simulink model "basic_DTC_model"  (R2024b)
settings: Solver=ode23tb  StartTime=0.0  StopTime=0.4  RelTol=1e-3
InitFcn:
  | pn = 4;
  | Ld = 8.5e-3;
  | Lq = 8.5e-3;
  | R = 1.2;
  | phi = 0.175;
  | J = 0.0008;
  | B = 0.000;
libraries: spsGroundLib x1, spsUniversalBridgeLib x1, spsPermanentMagnetSynchronousMachineLib x1, spsThreePhaseVIMeasurementLib x1, spsDCVoltageSourceLib x1, sps_lib x1

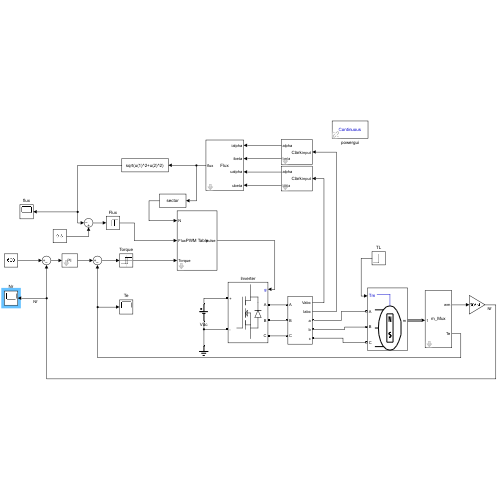
[thumbnail: Simulink's stored preview of the top-level diagram]
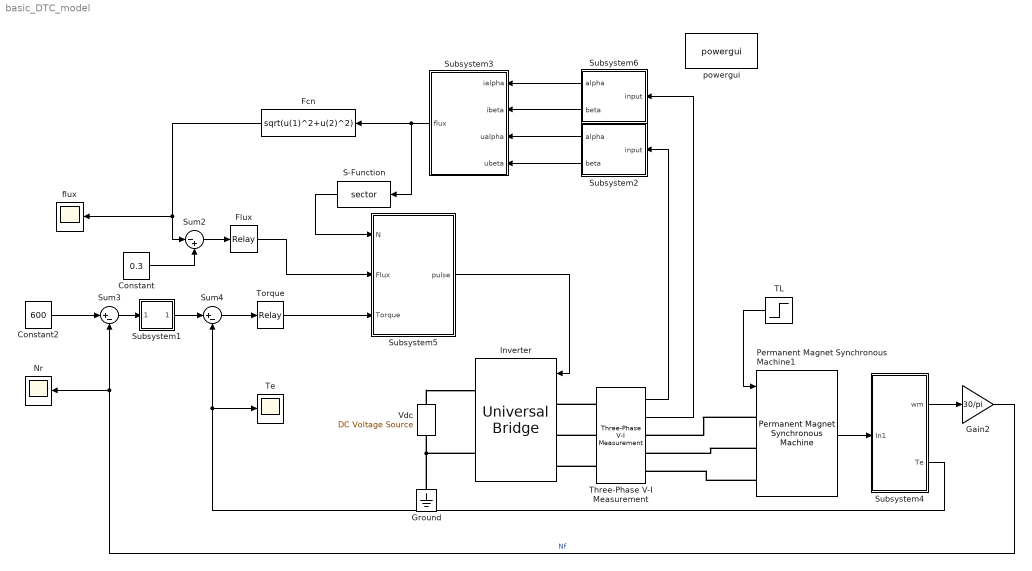
== system basic_DTC_model ==
  Constant : Constant  Value=0.3
  Constant2 : Constant  Value=600
  Fcn : Fcn  Expr=sqrt(u(1)^2+u(2)^2)
  Flux : Relay  OnSwitchValue=0.002  OffSwitchValue=-0.002
  Gain2 : Gain  Gain=30/pi
  Ground : spsGroundLib/Ground  LConnTagsString=a
  Inverter : spsUniversalBridgeLib/Universal Bridge  Arms=3  SnubberResistance=1e5  SnubberCapacitance=inf  Device=MOSFET / Diodes  Ron=1e-3  Lon=0  ForwardVoltages="[  0  0  ]"  ForwardVoltage=0  GTOparameters=[ 10e-6 , 20e-6 ]  IGBTparameters=[ 1e-6 , 2e-6 ]  Measurements=None  Measurements_2=None  converterType=Rectifier
  Nr : Scope
  Permanent Magnet Synchronous Machine1 : spsPermanentMagnetSynchronousMachineLib/Permanent Magnet Synchronous Machine  NbPhases=3  FluxDistribution=Sinusoidal  RotorType=Salient-pole  MechanicalLoad=Torque Tm  PresetModel=No  ShowDetailedParameters=on  MeasurementBus=off  Resistance=R  Inductance=8.5e-3  dqInductances=[Ld Lq]  La=0.000395  MachineConstant=Flux linkage established by magnets (V.s)  Flux=phi  VoltageCst=132.5525  TorqueCst=1.0962  Flat=120  Mechanical=[J B pn 0]  PolePairs=2  InitialConditions=[0,0, 0,0]  InitialConditions5ph=[0 0 0 0 0 0]  RefAngle=Aligned with phase A axis (original Park)  IterativeDiscreteModel=Trapezoidal non iterative  TsBlock=-1  TsPowergui=0
  S-Function : S-Function  FunctionName=sector  SFunctionModules='sector'  SFunctionDeploymentMode=off  EnableBusSupport=off
  Subsystem1 : Subsystem
  Subsystem2 : Subsystem
  Subsystem3 : Subsystem
  Subsystem4 : Subsystem
  Subsystem5 : Subsystem
  Subsystem6 : Subsystem
  Sum2 : Sum  Inputs=|-+
  Sum3 : Sum  Inputs=|+-
  Sum4 : Sum  Inputs=|+-
  TL : Step  Time=0.2  After=1.5  SampleTime=0
  Te : Scope
  Three-Phase V-I Measurement : spsThreePhaseVIMeasurementLib/Three-Phase V-I Measurement  VoltageMeasurement=phase-to-ground  SetLabelV=off  LabelV=Vabc  Vpu=off  VpuLL=off  CurrentMeasurement=yes  SetLabelI=off  LabelI=Iabc  Ipu=off  Pbase=100e6  Vbase=500e3  OutputType=Complex  PhasorSimulation=off  PSBequivalent=0
  Torque : Relay  OnSwitchValue=0.1  OffSwitchValue=-0.1
  Vdc : spsDCVoltageSourceLib/DC Voltage Source  Amplitude=311  Measurements=None
  flux : Scope
  powergui : sps_lib/powergui  Priority=1  SimulationMode=Continuous  SampleTime=10e-6  frequency=60  Iterations=50  frequencyindice=0  Pbase=100e6  ErrMax=1e-4  UnitsV=kV  UnitsW=MW  buscounter=0  FunctionMessages=off  echomessages=off  EnableUseOfTLC=off  CurrentSourceSwitches=off  DisableSnubberDevices=off  DisableRonSwitches=off  DisableVfSwitches=off  DisplayEquations=off  AutomaticDiscreteSolvers=off  SolverType=Tustin/Backward Euler (TBE)  Interpol=off  ExternalGateDelay=off  methode=off  Ts=100  x0status=blocks  SPID=on  SwTol=0  HookPort=off  NonlinearTolerance=1e-4  nMaxIteration=100  ContinueOnMaxIteration=off  RestoreLinks=warning  ResistiveCurrentMeasurement=off  Frange=[0:2:500]  Ylog=off  Xlog=on  ShowGrid=off  save=off  variable=ZData  structure=0  ZoomFFT=off  StartTime=0.0  cycles=1  DisplayStyle=1  fundamental=60  FreqAxis=off  MaxFrequency=1000  frequencyindicesteady=1  RmsSteady=1  display=off
  wires:
  TL/1 -> Permanent Magnet Synchronous Machine1/1
  Permanent Magnet Synchronous Machine1/1 -> Subsystem4/1(In1)
  Subsystem4/2(Te) -> Sum4/2, Te/1
  Subsystem5/1(pulse) -> Inverter/1
  Constant2/1 -> Sum3/1
  Sum3/1 -> Subsystem1/1(Input)
  Subsystem3/1(flux) -> S-Function/1, Fcn/1
  Constant/1 -> Sum2/2
  Fcn/1 -> flux/1, Sum2/1
  S-Function/1 -> Subsystem5/1(N)
  Sum2/1 -> Flux/1
  Flux/1 -> Subsystem5/2(Flux)
  Sum4/1 -> Torque/1
  Subsystem1/1(output) -> Sum4/1
  Torque/1 -> Subsystem5/3(Torque)
  Subsystem4/1(wm) -> Gain2/1
  Gain2/1 -> Sum3/2, Nr/1  "Nf"
  Three-Phase V-I Measurement/1 -> Subsystem2/1(input)
  Subsystem2/1(alpha) -> Subsystem3/3(ualpha)
  Subsystem2/2(beta) -> Subsystem3/4(ubeta)
  Subsystem6/2(beta) -> Subsystem3/2(ibeta)
  Subsystem6/1(alpha) -> Subsystem3/1(ialpha)
  Three-Phase V-I Measurement/2 -> Subsystem6/1(input)
  connections:
  Vdc/RConn1 -- Inverter/RConn1
  Inverter/RConn2 -- Ground/LConn1 -- Vdc/LConn1
  Three-Phase V-I Measurement/LConn1 -- Inverter/LConn1
  Three-Phase V-I Measurement/LConn2 -- Inverter/LConn2
  Three-Phase V-I Measurement/LConn3 -- Inverter/LConn3
  Permanent Magnet Synchronous Machine1/LConn1 -- Three-Phase V-I Measurement/RConn1
  Permanent Magnet Synchronous Machine1/LConn2 -- Three-Phase V-I Measurement/RConn2
  Permanent Magnet Synchronous Machine1/LConn3 -- Three-Phase V-I Measurement/RConn3

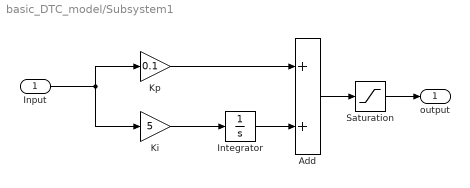
== system basic_DTC_model/Subsystem1 ==
  Input : Inport
  Add : Sum
  Integrator : Integrator
  Ki : Gain  Gain=5
  Kp : Gain  Gain=0.1
  Saturation : Saturate  UpperLimit=5  LowerLimit=-5
  output : Outport
  wires:
  Input/1 -> Ki/1, Kp/1
  Ki/1 -> Integrator/1
  Integrator/1 -> Add/2
  Kp/1 -> Add/1
  Add/1 -> Saturation/1
  Saturation/1 -> output/1

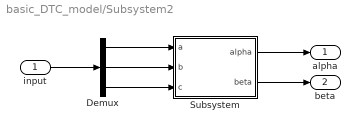
== system basic_DTC_model/Subsystem2 ==
  input : Inport
  Demux : Demux  Outputs=3
  Subsystem : Subsystem
  alpha : Outport
  beta : Outport  Port=2
  wires:
  input/1 -> Demux/1
  Demux/1 -> Subsystem/1(a)
  Demux/2 -> Subsystem/2(b)
  Demux/3 -> Subsystem/3(c)
  Subsystem/1(alpha) -> alpha/1
  Subsystem/2(beta) -> beta/1

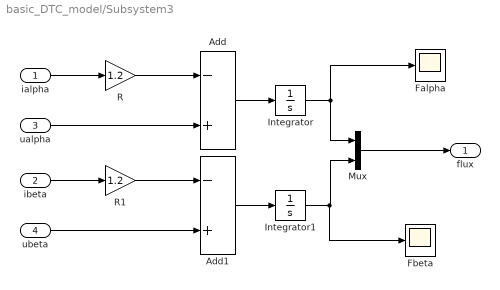
== system basic_DTC_model/Subsystem3 ==
  ialpha : Inport
  ibeta : Inport  Port=2
  ualpha : Inport  Port=3
  ubeta : Inport  Port=4
  Add : Sum  Inputs=-+
  Add1 : Sum  Inputs=-+
  Falpha : Scope
  Fbeta : Scope
  Integrator : Integrator
  Integrator1 : Integrator
  Mux : Mux  Inputs=2
  R : Gain  Gain=1.2
  R1 : Gain  Gain=1.2
  flux : Outport
  wires:
  ialpha/1 -> R/1
  ibeta/1 -> R1/1
  R/1 -> Add/1
  ualpha/1 -> Add/2
  Add/1 -> Integrator/1
  R1/1 -> Add1/1
  ubeta/1 -> Add1/2
  Add1/1 -> Integrator1/1
  Integrator/1 -> Falpha/1, Mux/1
  Integrator1/1 -> Fbeta/1, Mux/2
  Mux/1 -> flux/1

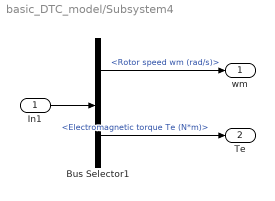
== system basic_DTC_model/Subsystem4 ==
  In1 : Inport
  Bus Selector1 : BusSelector  OutputSignals=Rotor speed wm (rad/s),Electromagnetic torque Te (N*m)
  wm : Outport
  Te : Outport  Port=2
  wires:
  In1/1 -> Bus Selector1/1
  Bus Selector1/1 -> wm/1  "<Rotor speed wm (rad/s)>"
  Bus Selector1/2 -> Te/1  "<Electromagnetic torque Te (N*m)>"

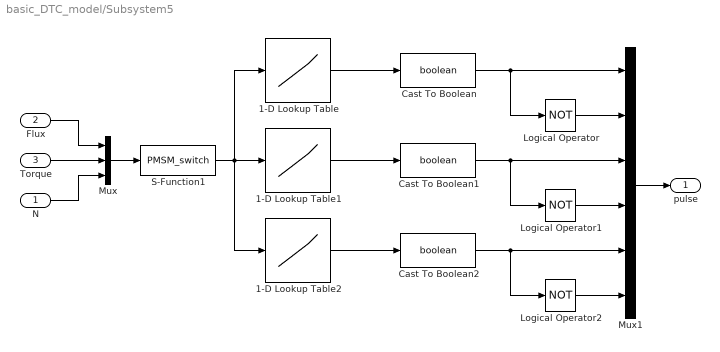
== system basic_DTC_model/Subsystem5 ==
  N : Inport
  Flux : Inport  Port=2
  Torque : Inport  Port=3
  1-D Lookup Table : Lookup_n-D  NumberOfTableDimensions=1  BreakpointsForDimension1=[1,2,3,4,5,6]  Table=[1,1,1,0,0,0]  InternalRulePriority=Speed  RndMeth=Simplest
  1-D Lookup Table1 : Lookup_n-D  NumberOfTableDimensions=1  BreakpointsForDimension1=[1,2,3,4,5,6]  Table=[1,0,0,1,1,0]  InternalRulePriority=Speed  RndMeth=Simplest
  1-D Lookup Table2 : Lookup_n-D  NumberOfTableDimensions=1  BreakpointsForDimension1=[1,2,3,4,5,6]  Table=[0,1,0,1,0,1]  InternalRulePriority=Speed  RndMeth=Simplest
  Cast To Boolean : DataTypeConversion  OutDataTypeStr=boolean  SaturateOnIntegerOverflow=off  RndMeth=Floor
  Cast To Boolean1 : DataTypeConversion  OutDataTypeStr=boolean  SaturateOnIntegerOverflow=off  RndMeth=Floor
  Cast To Boolean2 : DataTypeConversion  OutDataTypeStr=boolean  SaturateOnIntegerOverflow=off  RndMeth=Floor
  Logical Operator : Logic  Operator=NOT  AllPortsSameDT=off  OutDataTypeStr=boolean
  Logical Operator1 : Logic  Operator=NOT  AllPortsSameDT=off  OutDataTypeStr=boolean
  Logical Operator2 : Logic  Operator=NOT  AllPortsSameDT=off  OutDataTypeStr=boolean
  Mux : Mux  Inputs=3
  Mux1 : Mux  Inputs=6
  S-Function1 : S-Function  FunctionName=PMSM_switch  SFunctionModules='PMSM_switch'  SFunctionDeploymentMode=off  EnableBusSupport=off
  pulse : Outport
  wires:
  Torque/1 -> Mux/2
  Flux/1 -> Mux/1
  N/1 -> Mux/3
  Mux/1 -> S-Function1/1
  S-Function1/1 -> 1-D Lookup Table2/1, 1-D Lookup Table/1, 1-D Lookup Table1/1
  1-D Lookup Table/1 -> Cast To Boolean/1
  Cast To Boolean/1 -> Logical Operator/1, Mux1/1
  Logical Operator/1 -> Mux1/2
  Logical Operator1/1 -> Mux1/4
  1-D Lookup Table1/1 -> Cast To Boolean1/1
  Cast To Boolean1/1 -> Logical Operator1/1, Mux1/3
  Cast To Boolean2/1 -> Logical Operator2/1, Mux1/5
  Logical Operator2/1 -> Mux1/6
  1-D Lookup Table2/1 -> Cast To Boolean2/1
  Mux1/1 -> pulse/1

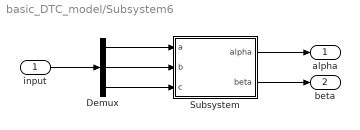
== system basic_DTC_model/Subsystem6 ==
  input : Inport
  Demux : Demux  Outputs=3
  Subsystem : Subsystem
  alpha : Outport
  beta : Outport  Port=2
  wires:
  input/1 -> Demux/1
  Demux/1 -> Subsystem/1(a)
  Demux/2 -> Subsystem/2(b)
  Demux/3 -> Subsystem/3(c)
  Subsystem/1(alpha) -> alpha/1
  Subsystem/2(beta) -> beta/1

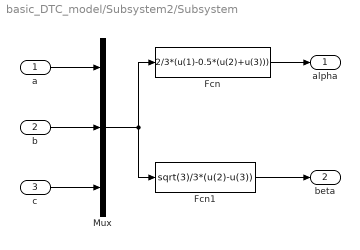
== system basic_DTC_model/Subsystem2/Subsystem ==
  a : Inport
  b : Inport  Port=2
  c : Inport  Port=3
  Fcn : Fcn  Expr=2/3*(u(1)-0.5*(u(2)+u(3)))
  Fcn1 : Fcn  Expr=sqrt(3)/3*(u(2)-u(3))
  Mux : Mux  Inputs=3
  alpha : Outport
  beta : Outport  Port=2
  wires:
  a/1 -> Mux/1
  b/1 -> Mux/2
  c/1 -> Mux/3
  Mux/1 -> Fcn/1, Fcn1/1
  Fcn/1 -> alpha/1
  Fcn1/1 -> beta/1

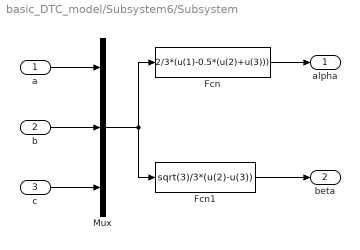
== system basic_DTC_model/Subsystem6/Subsystem ==
  a : Inport
  b : Inport  Port=2
  c : Inport  Port=3
  Fcn : Fcn  Expr=2/3*(u(1)-0.5*(u(2)+u(3)))
  Fcn1 : Fcn  Expr=sqrt(3)/3*(u(2)-u(3))
  Mux : Mux  Inputs=3
  alpha : Outport
  beta : Outport  Port=2
  wires:
  a/1 -> Mux/1
  b/1 -> Mux/2
  c/1 -> Mux/3
  Mux/1 -> Fcn/1, Fcn1/1
  Fcn/1 -> alpha/1
  Fcn1/1 -> beta/1
